simulink model "MyVhclOperator_RTW"  (Simulink 7.5)
settings: Solver=ode1  SolverMode=SingleTasking  StartTime=0.0  StopTime=inf  FixedStep=0.001  RelTol=1e-3
PreLoadFcn:
  | vehicle = 'Car'; if ~length(which('cmcmd')), cmenv; end
  | MyVhclOperator_RTW_bus
InitFcn:
  | vehicle = 'Car'; if ~length(which('cmcmd')), cmenv; end
  | MyVhclOperator_RTW_bus
undefined symbols (not defined in the file or in its folder): OperationFinished, Phase, SteerAng, VCBus
libraries: simulink x45
(part 2 of 3)

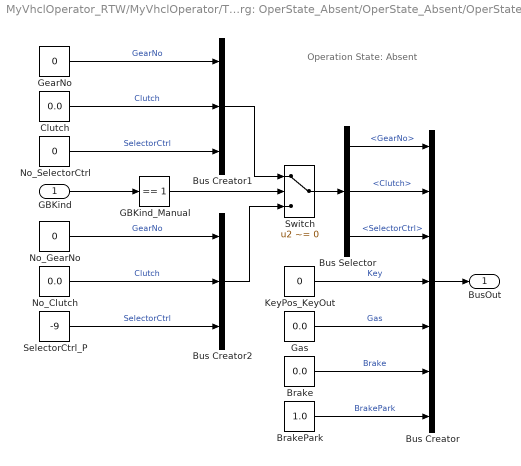
== system MyVhclOperator_RTW/MyVhclOperator/Trg: OperState_Absent/OperState_Absent/OperState: Absent ==
  note: Operation State:
      | Absent
  GBKind : Inport  OutDataType=fixdt(1, 16)  OutScaling=2^0
  Brake : Constant  Value=0.0  OutDataType=fixdt(1, 16)  OutScaling=2^0
  BrakePark : Constant  Value=1.0  OutDataType=fixdt(1, 16)  OutScaling=2^0
  Bus Creator : BusCreator  Inputs=7
  Bus Creator1 : BusCreator  Inputs=3
  Bus Creator2 : BusCreator  Inputs=3
  Bus Selector : BusSelector  OutputSignals=GearNo,Clutch,SelectorCtrl
  Clutch : Constant  Value=0.0  OutDataType=fixdt(1, 16)  OutScaling=2^0
  GBKind_Manual : simulink/Logic and Bit Operations/Compare To Constant  SystemSampleTime=-1  relop===  const=1  LogicOutDataTypeMode=uint8
  Gas : Constant  Value=0.0  OutDataType=fixdt(1, 16)  OutScaling=2^0
  GearNo : Constant  Value=0  OutDataType=fixdt(1, 16)  OutScaling=2^0
  KeyPos_KeyOut : Constant  Value=0  OutDataType=fixdt(1, 16)  OutScaling=2^0
  No_Clutch : Constant  Value=0.0  OutDataType=fixdt(1, 16)  OutScaling=2^0
  No_GearNo : Constant  Value=0  OutDataType=fixdt(1, 16)  OutScaling=2^0
  No_SelectorCtrl : Constant  Value=0  OutDataType=fixdt(1, 16)  OutScaling=2^0
  SelectorCtrl_P : Constant  Value=-9  OutDataType=fixdt(1, 16)  OutScaling=2^0
  Switch : Switch  Criteria=u2 ~= 0  OutDataType=fixdt(1, 16)  OutScaling=2^0
  BusOut : Outport  OutDataType=fixdt(1, 16)  OutScaling=2^0
  wires:
  GBKind_Manual/1 -> Switch/2
  GBKind/1 -> GBKind_Manual/1
  Bus Creator2/1 -> Switch/3
  SelectorCtrl_P/1 -> Bus Creator2/3  "SelectorCtrl"
  No_Clutch/1 -> Bus Creator2/2  "Clutch"
  No_GearNo/1 -> Bus Creator2/1  "GearNo"
  No_SelectorCtrl/1 -> Bus Creator1/3  "SelectorCtrl"
  Clutch/1 -> Bus Creator1/2  "Clutch"
  GearNo/1 -> Bus Creator1/1  "GearNo"
  Bus Creator1/1 -> Switch/1
  Switch/1 -> Bus Selector/1
  BrakePark/1 -> Bus Creator/7  "BrakePark"
  Brake/1 -> Bus Creator/6  "Brake"
  Gas/1 -> Bus Creator/5  "Gas"
  KeyPos_KeyOut/1 -> Bus Creator/4  "Key"
  Bus Selector/3 -> Bus Creator/3  "<SelectorCtrl>"
  Bus Selector/2 -> Bus Creator/2  "<Clutch>"
  Bus Selector/1 -> Bus Creator/1  "<GearNo>"
  Bus Creator/1 -> BusOut/1

== system MyVhclOperator_RTW/MyVhclOperator/Trg: OperState_Absent/OperState_Driving/Drive2Off ==
  note: Drive2Off
  BusIn : Inport  OutDataType=fixdt(1, 16)  OutScaling=2^0
  Active Brake : Subsystem  TreatAsAtomicUnit=on
  Brake to standstill? : Subsystem  TreatAsAtomicUnit=on
  Bus Selector : BusSelector  OutputSignals=Phase
  BusIn_Copy : InportShadow  Port=1  OutDataType=fixdt(1, 16)  OutScaling=2^0
  Key PowerOff : Subsystem  TreatAsAtomicUnit=on
  Merge : Merge  Inputs=5
  Switch Case : SwitchCase  CaseConditions={0,1,2,3,4}  ShowDefaultCase=off
  Wait for PowerOff : Subsystem  TreatAsAtomicUnit=on
  Wait until Standstill : Subsystem  TreatAsAtomicUnit=on
  BusOut : Outport  OutDataType=fixdt(1, 16)  OutScaling=2^0
  wires:
  Bus Selector/1 -> Switch Case/1  "<Phase>"
  Wait for PowerOff/1(BusOut) -> Merge/5
  Key PowerOff/1(BusOut) -> Merge/4
  Wait until Standstill/1(BusOut) -> Merge/3
  Active Brake/1(BusOut) -> Merge/2
  Brake to standstill?/1(BusOut) -> Merge/1
  BusIn_Copy/1 -> Brake to standstill?/1(BusIn), Active Brake/1(BusIn), Wait until Standstill/1(BusIn), Key PowerOff/1(BusIn), Wait for PowerOff/1(BusIn)
  Switch Case/5 -> Wait for PowerOff/Action
  Switch Case/4 -> Key PowerOff/Action
  Switch Case/3 -> Wait until Standstill/Action
  Merge/1 -> BusOut/1
  Switch Case/2 -> Active Brake/Action
  Switch Case/1 -> Brake to standstill?/Action
  BusIn/1 -> Bus Selector/1

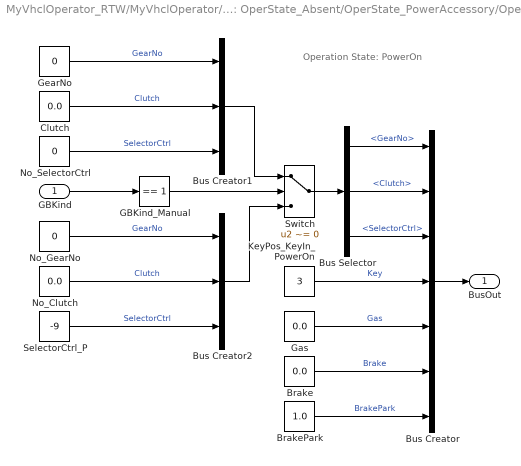
== system MyVhclOperator_RTW/MyVhclOperator/Trg: OperState_Absent/OperState_PowerAccessory/OperState: PowerOn ==
  note: Operation State:
      | PowerOn
  GBKind : Inport  OutDataType=fixdt(1, 16)  OutScaling=2^0
  Brake : Constant  Value=0.0  OutDataType=fixdt(1, 16)  OutScaling=2^0
  BrakePark : Constant  Value=1.0  OutDataType=fixdt(1, 16)  OutScaling=2^0
  Bus Creator : BusCreator  Inputs=7
  Bus Creator1 : BusCreator  Inputs=3
  Bus Creator2 : BusCreator  Inputs=3
  Bus Selector : BusSelector  OutputSignals=GearNo,Clutch,SelectorCtrl
  Clutch : Constant  Value=0.0  OutDataType=fixdt(1, 16)  OutScaling=2^0
  GBKind_Manual : simulink/Logic and Bit Operations/Compare To Constant  SystemSampleTime=-1  relop===  const=1  LogicOutDataTypeMode=uint8
  Gas : Constant  Value=0.0  OutDataType=fixdt(1, 16)  OutScaling=2^0
  GearNo : Constant  Value=0  OutDataType=fixdt(1, 16)  OutScaling=2^0
  KeyPos_KeyIn_PowerOn : Constant  Value=3  OutDataType=fixdt(1, 16)  OutScaling=2^0
  No_Clutch : Constant  Value=0.0  OutDataType=fixdt(1, 16)  OutScaling=2^0
  No_GearNo : Constant  Value=0  OutDataType=fixdt(1, 16)  OutScaling=2^0
  No_SelectorCtrl : Constant  Value=0  OutDataType=fixdt(1, 16)  OutScaling=2^0
  SelectorCtrl_P : Constant  Value=-9  OutDataType=fixdt(1, 16)  OutScaling=2^0
  Switch : Switch  Criteria=u2 ~= 0  OutDataType=fixdt(1, 16)  OutScaling=2^0
  BusOut : Outport  OutDataType=fixdt(1, 16)  OutScaling=2^0
  wires:
  GBKind_Manual/1 -> Switch/2
  GBKind/1 -> GBKind_Manual/1
  Bus Creator2/1 -> Switch/3
  SelectorCtrl_P/1 -> Bus Creator2/3  "SelectorCtrl"
  No_Clutch/1 -> Bus Creator2/2  "Clutch"
  No_GearNo/1 -> Bus Creator2/1  "GearNo"
  No_SelectorCtrl/1 -> Bus Creator1/3  "SelectorCtrl"
  Clutch/1 -> Bus Creator1/2  "Clutch"
  GearNo/1 -> Bus Creator1/1  "GearNo"
  Bus Creator1/1 -> Switch/1
  Switch/1 -> Bus Selector/1
  BrakePark/1 -> Bus Creator/7  "BrakePark"
  Brake/1 -> Bus Creator/6  "Brake"
  Gas/1 -> Bus Creator/5  "Gas"
  KeyPos_KeyIn_PowerOn/1 -> Bus Creator/4  "Key"
  Bus Selector/3 -> Bus Creator/3  "<SelectorCtrl>"
  Bus Selector/2 -> Bus Creator/2  "<Clutch>"
  Bus Selector/1 -> Bus Creator/1  "<GearNo>"
  Bus Creator/1 -> BusOut/1

== system MyVhclOperator_RTW/MyVhclOperator/Trg: OperState_Absent/OperState_PowerAccessory/SetOutputAndWait ==
  PhaseIn : Inport  OutDataType=fixdt(1, 16)  OutScaling=2^0
  Add : Sum  OutDataType=fixdt(1, 16)  OutScaling=2^-10
  Compare To Constant : simulink/Logic and Bit Operations/Compare To Constant  SystemSampleTime=-1  relop===  const=0  LogicOutDataTypeMode=uint8
  Constant : Constant  OutDataType=fixdt(1, 16)  OutScaling=2^0
  Switch : Switch  Criteria=u2 ~= 0  OutDataType=fixdt(1, 16)  OutScaling=2^0
  PhaseOut : Outport  OutDataType=fixdt(1, 16)  OutScaling=2^0
  wires:
  Constant/1 -> Add/1
  Add/1 -> Switch/1
  Compare To Constant/1 -> Switch/2
  PhaseIn/1 -> Add/2, Switch/3, Compare To Constant/1
  Switch/1 -> PhaseOut/1

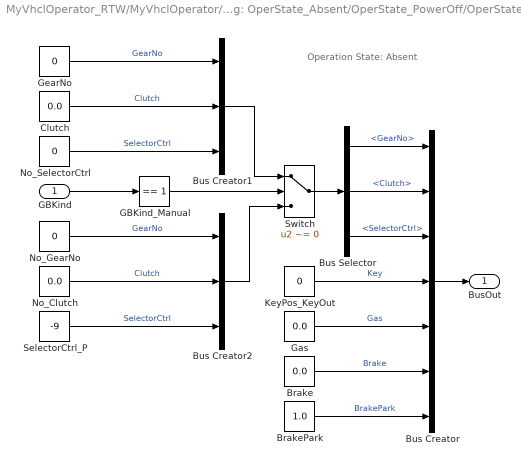
== system MyVhclOperator_RTW/MyVhclOperator/Trg: OperState_Absent/OperState_PowerOff/OperState: Absent ==
  note: Operation State:
      | Absent
  GBKind : Inport  OutDataType=fixdt(1, 16)  OutScaling=2^0
  Brake : Constant  Value=0.0  OutDataType=fixdt(1, 16)  OutScaling=2^0
  BrakePark : Constant  Value=1.0  OutDataType=fixdt(1, 16)  OutScaling=2^0
  Bus Creator : BusCreator  Inputs=7
  Bus Creator1 : BusCreator  Inputs=3
  Bus Creator2 : BusCreator  Inputs=3
  Bus Selector : BusSelector  OutputSignals=GearNo,Clutch,SelectorCtrl
  Clutch : Constant  Value=0.0  OutDataType=fixdt(1, 16)  OutScaling=2^0
  GBKind_Manual : simulink/Logic and Bit Operations/Compare To Constant  SystemSampleTime=-1  relop===  const=1  LogicOutDataTypeMode=uint8
  Gas : Constant  Value=0.0  OutDataType=fixdt(1, 16)  OutScaling=2^0
  GearNo : Constant  Value=0  OutDataType=fixdt(1, 16)  OutScaling=2^0
  KeyPos_KeyOut : Constant  Value=0  OutDataType=fixdt(1, 16)  OutScaling=2^0
  No_Clutch : Constant  Value=0.0  OutDataType=fixdt(1, 16)  OutScaling=2^0
  No_GearNo : Constant  Value=0  OutDataType=fixdt(1, 16)  OutScaling=2^0
  No_SelectorCtrl : Constant  Value=0  OutDataType=fixdt(1, 16)  OutScaling=2^0
  SelectorCtrl_P : Constant  Value=-9  OutDataType=fixdt(1, 16)  OutScaling=2^0
  Switch : Switch  Criteria=u2 ~= 0  OutDataType=fixdt(1, 16)  OutScaling=2^0
  BusOut : Outport  OutDataType=fixdt(1, 16)  OutScaling=2^0
  wires:
  GBKind_Manual/1 -> Switch/2
  GBKind/1 -> GBKind_Manual/1
  Bus Creator2/1 -> Switch/3
  SelectorCtrl_P/1 -> Bus Creator2/3  "SelectorCtrl"
  No_Clutch/1 -> Bus Creator2/2  "Clutch"
  No_GearNo/1 -> Bus Creator2/1  "GearNo"
  No_SelectorCtrl/1 -> Bus Creator1/3  "SelectorCtrl"
  Clutch/1 -> Bus Creator1/2  "Clutch"
  GearNo/1 -> Bus Creator1/1  "GearNo"
  Bus Creator1/1 -> Switch/1
  Switch/1 -> Bus Selector/1
  BrakePark/1 -> Bus Creator/7  "BrakePark"
  Brake/1 -> Bus Creator/6  "Brake"
  Gas/1 -> Bus Creator/5  "Gas"
  KeyPos_KeyOut/1 -> Bus Creator/4  "Key"
  Bus Selector/3 -> Bus Creator/3  "<SelectorCtrl>"
  Bus Selector/2 -> Bus Creator/2  "<Clutch>"
  Bus Selector/1 -> Bus Creator/1  "<GearNo>"
  Bus Creator/1 -> BusOut/1

== system MyVhclOperator_RTW/MyVhclOperator/Trg: OperState_Absent/OperState_PowerOff/SetOutputAndWait ==
  PhaseIn : Inport  OutDataType=fixdt(1, 16)  OutScaling=2^0
  Add : Sum  OutDataType=fixdt(1, 16)  OutScaling=2^-10
  Compare To Constant : simulink/Logic and Bit Operations/Compare To Constant  SystemSampleTime=-1  relop===  const=0  LogicOutDataTypeMode=uint8
  Constant : Constant  OutDataType=fixdt(1, 16)  OutScaling=2^0
  Switch : Switch  Criteria=u2 ~= 0  OutDataType=fixdt(1, 16)  OutScaling=2^0
  PhaseOut : Outport  OutDataType=fixdt(1, 16)  OutScaling=2^0
  wires:
  Constant/1 -> Add/1
  Add/1 -> Switch/1
  Compare To Constant/1 -> Switch/2
  PhaseIn/1 -> Add/2, Switch/3, Compare To Constant/1
  Switch/1 -> PhaseOut/1

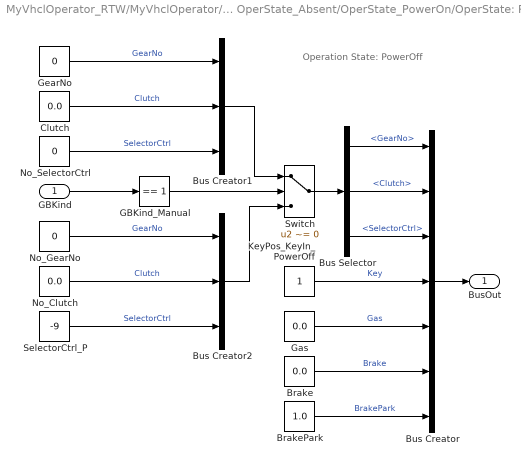
== system MyVhclOperator_RTW/MyVhclOperator/Trg: OperState_Absent/OperState_PowerOn/OperState: PowerOff ==
  note: Operation State:
      | PowerOff
  GBKind : Inport  OutDataType=fixdt(1, 16)  OutScaling=2^0
  Brake : Constant  Value=0.0  OutDataType=fixdt(1, 16)  OutScaling=2^0
  BrakePark : Constant  Value=1.0  OutDataType=fixdt(1, 16)  OutScaling=2^0
  Bus Creator : BusCreator  Inputs=7
  Bus Creator1 : BusCreator  Inputs=3
  Bus Creator2 : BusCreator  Inputs=3
  Bus Selector : BusSelector  OutputSignals=GearNo,Clutch,SelectorCtrl
  Clutch : Constant  Value=0.0  OutDataType=fixdt(1, 16)  OutScaling=2^0
  GBKind_Manual : simulink/Logic and Bit Operations/Compare To Constant  SystemSampleTime=-1  relop===  const=1  LogicOutDataTypeMode=uint8
  Gas : Constant  Value=0.0  OutDataType=fixdt(1, 16)  OutScaling=2^0
  GearNo : Constant  Value=0  OutDataType=fixdt(1, 16)  OutScaling=2^0
  KeyPos_KeyIn_PowerOff : Constant  OutDataType=fixdt(1, 16)  OutScaling=2^0
  No_Clutch : Constant  Value=0.0  OutDataType=fixdt(1, 16)  OutScaling=2^0
  No_GearNo : Constant  Value=0  OutDataType=fixdt(1, 16)  OutScaling=2^0
  No_SelectorCtrl : Constant  Value=0  OutDataType=fixdt(1, 16)  OutScaling=2^0
  SelectorCtrl_P : Constant  Value=-9  OutDataType=fixdt(1, 16)  OutScaling=2^0
  Switch : Switch  Criteria=u2 ~= 0  OutDataType=fixdt(1, 16)  OutScaling=2^0
  BusOut : Outport  OutDataType=fixdt(1, 16)  OutScaling=2^0
  wires:
  GBKind_Manual/1 -> Switch/2
  GBKind/1 -> GBKind_Manual/1
  Bus Creator2/1 -> Switch/3
  SelectorCtrl_P/1 -> Bus Creator2/3  "SelectorCtrl"
  No_Clutch/1 -> Bus Creator2/2  "Clutch"
  No_GearNo/1 -> Bus Creator2/1  "GearNo"
  No_SelectorCtrl/1 -> Bus Creator1/3  "SelectorCtrl"
  Clutch/1 -> Bus Creator1/2  "Clutch"
  GearNo/1 -> Bus Creator1/1  "GearNo"
  Bus Creator1/1 -> Switch/1
  Switch/1 -> Bus Selector/1
  BrakePark/1 -> Bus Creator/7  "BrakePark"
  Brake/1 -> Bus Creator/6  "Brake"
  Gas/1 -> Bus Creator/5  "Gas"
  KeyPos_KeyIn_PowerOff/1 -> Bus Creator/4  "Key"
  Bus Selector/3 -> Bus Creator/3  "<SelectorCtrl>"
  Bus Selector/2 -> Bus Creator/2  "<Clutch>"
  Bus Selector/1 -> Bus Creator/1  "<GearNo>"
  Bus Creator/1 -> BusOut/1

== system MyVhclOperator_RTW/MyVhclOperator/Trg: OperState_Absent/OperState_PowerOn/SetOutputAndWait ==
  PhaseIn : Inport  OutDataType=fixdt(1, 16)  OutScaling=2^0
  Add : Sum  OutDataType=fixdt(1, 16)  OutScaling=2^-10
  Compare To Constant : simulink/Logic and Bit Operations/Compare To Constant  SystemSampleTime=-1  relop===  const=0  LogicOutDataTypeMode=uint8
  Constant : Constant  OutDataType=fixdt(1, 16)  OutScaling=2^0
  Switch : Switch  Criteria=u2 ~= 0  OutDataType=fixdt(1, 16)  OutScaling=2^0
  PhaseOut : Outport  OutDataType=fixdt(1, 16)  OutScaling=2^0
  wires:
  Switch/1 -> PhaseOut/1
  PhaseIn/1 -> Compare To Constant/1, Switch/3, Add/2
  Compare To Constant/1 -> Switch/2
  Add/1 -> Switch/1
  Constant/1 -> Add/1

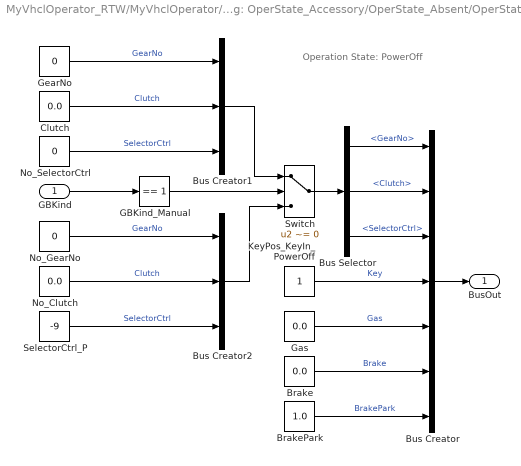
== system MyVhclOperator_RTW/MyVhclOperator/Trg: OperState_Accessory/OperState_Absent/OperState: PowerOff ==
  note: Operation State:
      | PowerOff
  GBKind : Inport  OutDataType=fixdt(1, 16)  OutScaling=2^0
  Brake : Constant  Value=0.0  OutDataType=fixdt(1, 16)  OutScaling=2^0
  BrakePark : Constant  Value=1.0  OutDataType=fixdt(1, 16)  OutScaling=2^0
  Bus Creator : BusCreator  Inputs=7
  Bus Creator1 : BusCreator  Inputs=3
  Bus Creator2 : BusCreator  Inputs=3
  Bus Selector : BusSelector  OutputSignals=GearNo,Clutch,SelectorCtrl
  Clutch : Constant  Value=0.0  OutDataType=fixdt(1, 16)  OutScaling=2^0
  GBKind_Manual : simulink/Logic and Bit Operations/Compare To Constant  SystemSampleTime=-1  relop===  const=1  LogicOutDataTypeMode=uint8
  Gas : Constant  Value=0.0  OutDataType=fixdt(1, 16)  OutScaling=2^0
  GearNo : Constant  Value=0  OutDataType=fixdt(1, 16)  OutScaling=2^0
  KeyPos_KeyIn_PowerOff : Constant  OutDataType=fixdt(1, 16)  OutScaling=2^0
  No_Clutch : Constant  Value=0.0  OutDataType=fixdt(1, 16)  OutScaling=2^0
  No_GearNo : Constant  Value=0  OutDataType=fixdt(1, 16)  OutScaling=2^0
  No_SelectorCtrl : Constant  Value=0  OutDataType=fixdt(1, 16)  OutScaling=2^0
  SelectorCtrl_P : Constant  Value=-9  OutDataType=fixdt(1, 16)  OutScaling=2^0
  Switch : Switch  Criteria=u2 ~= 0  OutDataType=fixdt(1, 16)  OutScaling=2^0
  BusOut : Outport  OutDataType=fixdt(1, 16)  OutScaling=2^0
  wires:
  Bus Creator/1 -> BusOut/1
  Bus Selector/1 -> Bus Creator/1  "<GearNo>"
  Bus Selector/2 -> Bus Creator/2  "<Clutch>"
  Bus Selector/3 -> Bus Creator/3  "<SelectorCtrl>"
  KeyPos_KeyIn_PowerOff/1 -> Bus Creator/4  "Key"
  Gas/1 -> Bus Creator/5  "Gas"
  Brake/1 -> Bus Creator/6  "Brake"
  BrakePark/1 -> Bus Creator/7  "BrakePark"
  Switch/1 -> Bus Selector/1
  Bus Creator1/1 -> Switch/1
  GearNo/1 -> Bus Creator1/1  "GearNo"
  Clutch/1 -> Bus Creator1/2  "Clutch"
  No_SelectorCtrl/1 -> Bus Creator1/3  "SelectorCtrl"
  No_GearNo/1 -> Bus Creator2/1  "GearNo"
  No_Clutch/1 -> Bus Creator2/2  "Clutch"
  SelectorCtrl_P/1 -> Bus Creator2/3  "SelectorCtrl"
  Bus Creator2/1 -> Switch/3
  GBKind/1 -> GBKind_Manual/1
  GBKind_Manual/1 -> Switch/2

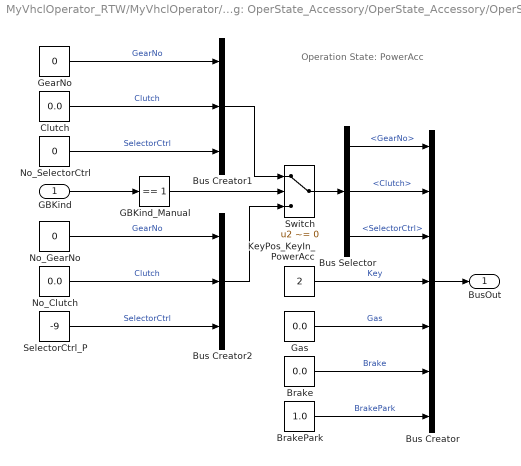
== system MyVhclOperator_RTW/MyVhclOperator/Trg: OperState_Accessory/OperState_Accessory/OperState: PowerAcc ==
  note: Operation State:
      | PowerAcc
  GBKind : Inport  OutDataType=fixdt(1, 16)  OutScaling=2^0
  Brake : Constant  Value=0.0  OutDataType=fixdt(1, 16)  OutScaling=2^0
  BrakePark : Constant  Value=1.0  OutDataType=fixdt(1, 16)  OutScaling=2^0
  Bus Creator : BusCreator  Inputs=7
  Bus Creator1 : BusCreator  Inputs=3
  Bus Creator2 : BusCreator  Inputs=3
  Bus Selector : BusSelector  OutputSignals=GearNo,Clutch,SelectorCtrl
  Clutch : Constant  Value=0.0  OutDataType=fixdt(1, 16)  OutScaling=2^0
  GBKind_Manual : simulink/Logic and Bit Operations/Compare To Constant  SystemSampleTime=-1  relop===  const=1  LogicOutDataTypeMode=uint8
  Gas : Constant  Value=0.0  OutDataType=fixdt(1, 16)  OutScaling=2^0
  GearNo : Constant  Value=0  OutDataType=fixdt(1, 16)  OutScaling=2^0
  KeyPos_KeyIn_PowerAcc : Constant  Value=2  OutDataType=fixdt(1, 16)  OutScaling=2^0
  No_Clutch : Constant  Value=0.0  OutDataType=fixdt(1, 16)  OutScaling=2^0
  No_GearNo : Constant  Value=0  OutDataType=fixdt(1, 16)  OutScaling=2^0
  No_SelectorCtrl : Constant  Value=0  OutDataType=fixdt(1, 16)  OutScaling=2^0
  SelectorCtrl_P : Constant  Value=-9  OutDataType=fixdt(1, 16)  OutScaling=2^0
  Switch : Switch  Criteria=u2 ~= 0  OutDataType=fixdt(1, 16)  OutScaling=2^0
  BusOut : Outport  OutDataType=fixdt(1, 16)  OutScaling=2^0
  wires:
  GBKind_Manual/1 -> Switch/2
  GBKind/1 -> GBKind_Manual/1
  Bus Creator2/1 -> Switch/3
  SelectorCtrl_P/1 -> Bus Creator2/3  "SelectorCtrl"
  No_Clutch/1 -> Bus Creator2/2  "Clutch"
  No_GearNo/1 -> Bus Creator2/1  "GearNo"
  No_SelectorCtrl/1 -> Bus Creator1/3  "SelectorCtrl"
  Clutch/1 -> Bus Creator1/2  "Clutch"
  GearNo/1 -> Bus Creator1/1  "GearNo"
  Bus Creator1/1 -> Switch/1
  Switch/1 -> Bus Selector/1
  BrakePark/1 -> Bus Creator/7  "BrakePark"
  Brake/1 -> Bus Creator/6  "Brake"
  Gas/1 -> Bus Creator/5  "Gas"
  KeyPos_KeyIn_PowerAcc/1 -> Bus Creator/4  "Key"
  Bus Selector/3 -> Bus Creator/3  "<SelectorCtrl>"
  Bus Selector/2 -> Bus Creator/2  "<Clutch>"
  Bus Selector/1 -> Bus Creator/1  "<GearNo>"
  Bus Creator/1 -> BusOut/1

== system MyVhclOperator_RTW/MyVhclOperator/Trg: OperState_Accessory/OperState_Driving/Drive2Off ==
  note: Drive2Off
  BusIn : Inport  OutDataType=fixdt(1, 16)  OutScaling=2^0
  Active Brake : Subsystem  TreatAsAtomicUnit=on
  Brake to standstill? : Subsystem  TreatAsAtomicUnit=on
  Bus Selector : BusSelector  OutputSignals=Phase
  BusIn_Copy : InportShadow  Port=1  OutDataType=fixdt(1, 16)  OutScaling=2^0
  Key PowerOff : Subsystem  TreatAsAtomicUnit=on
  Merge : Merge  Inputs=5
  Switch Case : SwitchCase  CaseConditions={0,1,2,3,4}  ShowDefaultCase=off
  Wait for PowerOff : Subsystem  TreatAsAtomicUnit=on
  Wait until Standstill : Subsystem  TreatAsAtomicUnit=on
  BusOut : Outport  OutDataType=fixdt(1, 16)  OutScaling=2^0
  wires:
  Bus Selector/1 -> Switch Case/1  "<Phase>"
  Wait for PowerOff/1(BusOut) -> Merge/5
  Key PowerOff/1(BusOut) -> Merge/4
  Wait until Standstill/1(BusOut) -> Merge/3
  Active Brake/1(BusOut) -> Merge/2
  Brake to standstill?/1(BusOut) -> Merge/1
  BusIn_Copy/1 -> Brake to standstill?/1(BusIn), Active Brake/1(BusIn), Wait until Standstill/1(BusIn), Key PowerOff/1(BusIn), Wait for PowerOff/1(BusIn)
  Switch Case/5 -> Wait for PowerOff/Action
  Switch Case/4 -> Key PowerOff/Action
  Switch Case/3 -> Wait until Standstill/Action
  Merge/1 -> BusOut/1
  Switch Case/2 -> Active Brake/Action
  Switch Case/1 -> Brake to standstill?/Action
  BusIn/1 -> Bus Selector/1

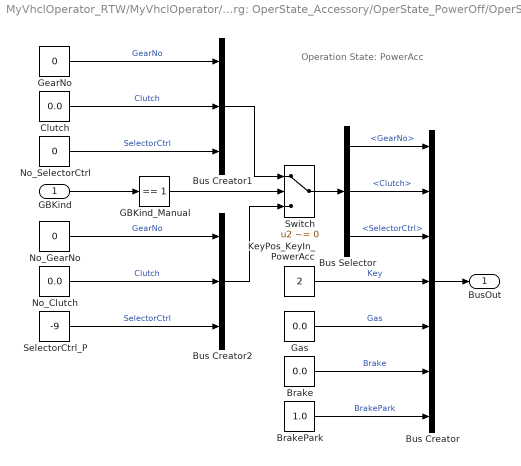
== system MyVhclOperator_RTW/MyVhclOperator/Trg: OperState_Accessory/OperState_PowerOff/OperState: PowerAcc ==
  note: Operation State:
      | PowerAcc
  GBKind : Inport  OutDataType=fixdt(1, 16)  OutScaling=2^0
  Brake : Constant  Value=0.0  OutDataType=fixdt(1, 16)  OutScaling=2^0
  BrakePark : Constant  Value=1.0  OutDataType=fixdt(1, 16)  OutScaling=2^0
  Bus Creator : BusCreator  Inputs=7
  Bus Creator1 : BusCreator  Inputs=3
  Bus Creator2 : BusCreator  Inputs=3
  Bus Selector : BusSelector  OutputSignals=GearNo,Clutch,SelectorCtrl
  Clutch : Constant  Value=0.0  OutDataType=fixdt(1, 16)  OutScaling=2^0
  GBKind_Manual : simulink/Logic and Bit Operations/Compare To Constant  SystemSampleTime=-1  relop===  const=1  LogicOutDataTypeMode=uint8
  Gas : Constant  Value=0.0  OutDataType=fixdt(1, 16)  OutScaling=2^0
  GearNo : Constant  Value=0  OutDataType=fixdt(1, 16)  OutScaling=2^0
  KeyPos_KeyIn_PowerAcc : Constant  Value=2  OutDataType=fixdt(1, 16)  OutScaling=2^0
  No_Clutch : Constant  Value=0.0  OutDataType=fixdt(1, 16)  OutScaling=2^0
  No_GearNo : Constant  Value=0  OutDataType=fixdt(1, 16)  OutScaling=2^0
  No_SelectorCtrl : Constant  Value=0  OutDataType=fixdt(1, 16)  OutScaling=2^0
  SelectorCtrl_P : Constant  Value=-9  OutDataType=fixdt(1, 16)  OutScaling=2^0
  Switch : Switch  Criteria=u2 ~= 0  OutDataType=fixdt(1, 16)  OutScaling=2^0
  BusOut : Outport  OutDataType=fixdt(1, 16)  OutScaling=2^0
  wires:
  GBKind_Manual/1 -> Switch/2
  GBKind/1 -> GBKind_Manual/1
  Bus Creator2/1 -> Switch/3
  SelectorCtrl_P/1 -> Bus Creator2/3  "SelectorCtrl"
  No_Clutch/1 -> Bus Creator2/2  "Clutch"
  No_GearNo/1 -> Bus Creator2/1  "GearNo"
  No_SelectorCtrl/1 -> Bus Creator1/3  "SelectorCtrl"
  Clutch/1 -> Bus Creator1/2  "Clutch"
  GearNo/1 -> Bus Creator1/1  "GearNo"
  Bus Creator1/1 -> Switch/1
  Switch/1 -> Bus Selector/1
  BrakePark/1 -> Bus Creator/7  "BrakePark"
  Brake/1 -> Bus Creator/6  "Brake"
  Gas/1 -> Bus Creator/5  "Gas"
  KeyPos_KeyIn_PowerAcc/1 -> Bus Creator/4  "Key"
  Bus Selector/3 -> Bus Creator/3  "<SelectorCtrl>"
  Bus Selector/2 -> Bus Creator/2  "<Clutch>"
  Bus Selector/1 -> Bus Creator/1  "<GearNo>"
  Bus Creator/1 -> BusOut/1

== system MyVhclOperator_RTW/MyVhclOperator/Trg: OperState_Accessory/OperState_PowerOff/SetOutputAndWait ==
  PhaseIn : Inport  OutDataType=fixdt(1, 16)  OutScaling=2^0
  Add : Sum  OutDataType=fixdt(1, 16)  OutScaling=2^-10
  Compare To Constant : simulink/Logic and Bit Operations/Compare To Constant  SystemSampleTime=-1  relop===  const=0  LogicOutDataTypeMode=uint8
  Constant : Constant  OutDataType=fixdt(1, 16)  OutScaling=2^0
  Switch : Switch  Criteria=u2 ~= 0  OutDataType=fixdt(1, 16)  OutScaling=2^0
  PhaseOut : Outport  OutDataType=fixdt(1, 16)  OutScaling=2^0
  wires:
  Switch/1 -> PhaseOut/1
  PhaseIn/1 -> Compare To Constant/1, Switch/3, Add/2
  Compare To Constant/1 -> Switch/2
  Add/1 -> Switch/1
  Constant/1 -> Add/1

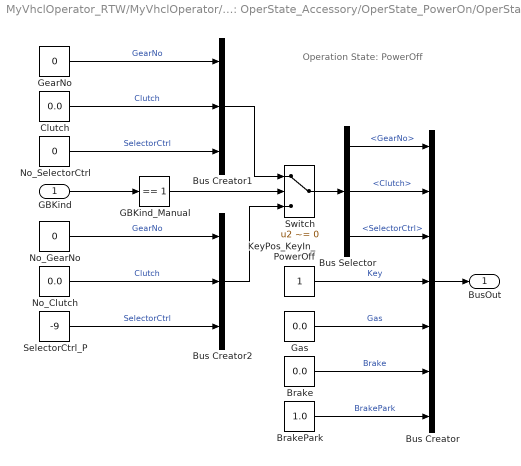
== system MyVhclOperator_RTW/MyVhclOperator/Trg: OperState_Accessory/OperState_PowerOn/OperState: PowerOff ==
  note: Operation State:
      | PowerOff
  GBKind : Inport  OutDataType=fixdt(1, 16)  OutScaling=2^0
  Brake : Constant  Value=0.0  OutDataType=fixdt(1, 16)  OutScaling=2^0
  BrakePark : Constant  Value=1.0  OutDataType=fixdt(1, 16)  OutScaling=2^0
  Bus Creator : BusCreator  Inputs=7
  Bus Creator1 : BusCreator  Inputs=3
  Bus Creator2 : BusCreator  Inputs=3
  Bus Selector : BusSelector  OutputSignals=GearNo,Clutch,SelectorCtrl
  Clutch : Constant  Value=0.0  OutDataType=fixdt(1, 16)  OutScaling=2^0
  GBKind_Manual : simulink/Logic and Bit Operations/Compare To Constant  SystemSampleTime=-1  relop===  const=1  LogicOutDataTypeMode=uint8
  Gas : Constant  Value=0.0  OutDataType=fixdt(1, 16)  OutScaling=2^0
  GearNo : Constant  Value=0  OutDataType=fixdt(1, 16)  OutScaling=2^0
  KeyPos_KeyIn_PowerOff : Constant  OutDataType=fixdt(1, 16)  OutScaling=2^0
  No_Clutch : Constant  Value=0.0  OutDataType=fixdt(1, 16)  OutScaling=2^0
  No_GearNo : Constant  Value=0  OutDataType=fixdt(1, 16)  OutScaling=2^0
  No_SelectorCtrl : Constant  Value=0  OutDataType=fixdt(1, 16)  OutScaling=2^0
  SelectorCtrl_P : Constant  Value=-9  OutDataType=fixdt(1, 16)  OutScaling=2^0
  Switch : Switch  Criteria=u2 ~= 0  OutDataType=fixdt(1, 16)  OutScaling=2^0
  BusOut : Outport  OutDataType=fixdt(1, 16)  OutScaling=2^0
  wires:
  GBKind_Manual/1 -> Switch/2
  GBKind/1 -> GBKind_Manual/1
  Bus Creator2/1 -> Switch/3
  SelectorCtrl_P/1 -> Bus Creator2/3  "SelectorCtrl"
  No_Clutch/1 -> Bus Creator2/2  "Clutch"
  No_GearNo/1 -> Bus Creator2/1  "GearNo"
  No_SelectorCtrl/1 -> Bus Creator1/3  "SelectorCtrl"
  Clutch/1 -> Bus Creator1/2  "Clutch"
  GearNo/1 -> Bus Creator1/1  "GearNo"
  Bus Creator1/1 -> Switch/1
  Switch/1 -> Bus Selector/1
  BrakePark/1 -> Bus Creator/7  "BrakePark"
  Brake/1 -> Bus Creator/6  "Brake"
  Gas/1 -> Bus Creator/5  "Gas"
  KeyPos_KeyIn_PowerOff/1 -> Bus Creator/4  "Key"
  Bus Selector/3 -> Bus Creator/3  "<SelectorCtrl>"
  Bus Selector/2 -> Bus Creator/2  "<Clutch>"
  Bus Selector/1 -> Bus Creator/1  "<GearNo>"
  Bus Creator/1 -> BusOut/1

== system MyVhclOperator_RTW/MyVhclOperator/Trg: OperState_Accessory/OperState_PowerOn/SetOutputAndWait ==
  PhaseIn : Inport  OutDataType=fixdt(1, 16)  OutScaling=2^0
  Add : Sum  OutDataType=fixdt(1, 16)  OutScaling=2^-10
  Compare To Constant : simulink/Logic and Bit Operations/Compare To Constant  SystemSampleTime=-1  relop===  const=0  LogicOutDataTypeMode=uint8
  Constant : Constant  OutDataType=fixdt(1, 16)  OutScaling=2^0
  Switch : Switch  Criteria=u2 ~= 0  OutDataType=fixdt(1, 16)  OutScaling=2^0
  PhaseOut : Outport  OutDataType=fixdt(1, 16)  OutScaling=2^0
  wires:
  Switch/1 -> PhaseOut/1
  PhaseIn/1 -> Compare To Constant/1, Switch/3, Add/2
  Compare To Constant/1 -> Switch/2
  Add/1 -> Switch/1
  Constant/1 -> Add/1

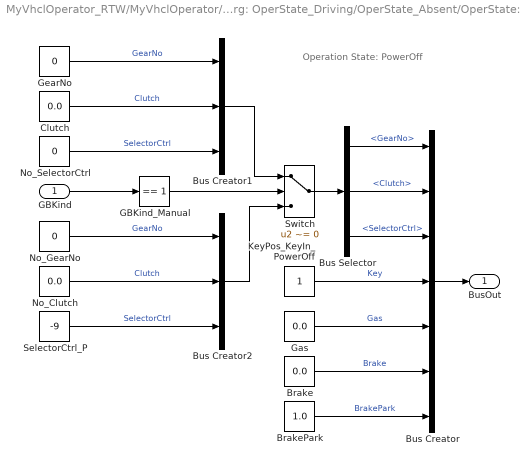
== system MyVhclOperator_RTW/MyVhclOperator/Trg: OperState_Driving/OperState_Absent/OperState: PowerOff ==
  note: Operation State:
      | PowerOff
  GBKind : Inport  OutDataType=fixdt(1, 16)  OutScaling=2^0
  Brake : Constant  Value=0.0  OutDataType=fixdt(1, 16)  OutScaling=2^0
  BrakePark : Constant  Value=1.0  OutDataType=fixdt(1, 16)  OutScaling=2^0
  Bus Creator : BusCreator  Inputs=7
  Bus Creator1 : BusCreator  Inputs=3
  Bus Creator2 : BusCreator  Inputs=3
  Bus Selector : BusSelector  OutputSignals=GearNo,Clutch,SelectorCtrl
  Clutch : Constant  Value=0.0  OutDataType=fixdt(1, 16)  OutScaling=2^0
  GBKind_Manual : simulink/Logic and Bit Operations/Compare To Constant  SystemSampleTime=-1  relop===  const=1  LogicOutDataTypeMode=uint8
  Gas : Constant  Value=0.0  OutDataType=fixdt(1, 16)  OutScaling=2^0
  GearNo : Constant  Value=0  OutDataType=fixdt(1, 16)  OutScaling=2^0
  KeyPos_KeyIn_PowerOff : Constant  OutDataType=fixdt(1, 16)  OutScaling=2^0
  No_Clutch : Constant  Value=0.0  OutDataType=fixdt(1, 16)  OutScaling=2^0
  No_GearNo : Constant  Value=0  OutDataType=fixdt(1, 16)  OutScaling=2^0
  No_SelectorCtrl : Constant  Value=0  OutDataType=fixdt(1, 16)  OutScaling=2^0
  SelectorCtrl_P : Constant  Value=-9  OutDataType=fixdt(1, 16)  OutScaling=2^0
  Switch : Switch  Criteria=u2 ~= 0  OutDataType=fixdt(1, 16)  OutScaling=2^0
  BusOut : Outport  OutDataType=fixdt(1, 16)  OutScaling=2^0
  wires:
  GBKind_Manual/1 -> Switch/2
  GBKind/1 -> GBKind_Manual/1
  Bus Creator2/1 -> Switch/3
  SelectorCtrl_P/1 -> Bus Creator2/3  "SelectorCtrl"
  No_Clutch/1 -> Bus Creator2/2  "Clutch"
  No_GearNo/1 -> Bus Creator2/1  "GearNo"
  No_SelectorCtrl/1 -> Bus Creator1/3  "SelectorCtrl"
  Clutch/1 -> Bus Creator1/2  "Clutch"
  GearNo/1 -> Bus Creator1/1  "GearNo"
  Bus Creator1/1 -> Switch/1
  Switch/1 -> Bus Selector/1
  BrakePark/1 -> Bus Creator/7  "BrakePark"
  Brake/1 -> Bus Creator/6  "Brake"
  Gas/1 -> Bus Creator/5  "Gas"
  KeyPos_KeyIn_PowerOff/1 -> Bus Creator/4  "Key"
  Bus Selector/3 -> Bus Creator/3  "<SelectorCtrl>"
  Bus Selector/2 -> Bus Creator/2  "<Clutch>"
  Bus Selector/1 -> Bus Creator/1  "<GearNo>"
  Bus Creator/1 -> BusOut/1

== system MyVhclOperator_RTW/MyVhclOperator/Trg: OperState_Driving/OperState_Driving/OperState: Driving ==
  note: Operation State:
      | Driving
  GBKind : Inport  OutDataType=fixdt(1, 16)  OutScaling=2^0
  Brake : Constant  Value=0.0  OutDataType=fixdt(1, 16)  OutScaling=2^0
  BrakePark : Constant  Value=0.0  OutDataType=fixdt(1, 16)  OutScaling=2^0
  Bus Creator : BusCreator  Inputs=7
  Bus Creator1 : BusCreator  Inputs=3
  Bus Creator2 : BusCreator  Inputs=3
  Bus Selector : BusSelector  OutputSignals=GearNo,Clutch,SelectorCtrl
  Clutch : Constant  Value=1.0  OutDataType=fixdt(1, 16)  OutScaling=2^0
  GBKind_Manual : simulink/Logic and Bit Operations/Compare To Constant  SystemSampleTime=-1  relop===  const=1  LogicOutDataTypeMode=uint8
  Gas : Constant  Value=0.0  OutDataType=fixdt(1, 16)  OutScaling=2^0
  GearNo : Constant  OutDataType=fixdt(1, 16)  OutScaling=2^0
  KeyPos_KeyIn_PowerOn : Constant  Value=3  OutDataType=fixdt(1, 16)  OutScaling=2^0
  No_Clutch : Constant  Value=0.0  OutDataType=fixdt(1, 16)  OutScaling=2^0
  No_GearNo : Constant  Value=0  OutDataType=fixdt(1, 16)  OutScaling=2^0
  No_SelectorCtrl : Constant  Value=0  OutDataType=fixdt(1, 16)  OutScaling=2^0
  SelectorCtrl_D : Constant  OutDataType=fixdt(1, 16)  OutScaling=2^0
  Switch : Switch  Criteria=u2 ~= 0  OutDataType=fixdt(1, 16)  OutScaling=2^0
  BusOut : Outport  OutDataType=fixdt(1, 16)  OutScaling=2^0
  wires:
  GBKind_Manual/1 -> Switch/2
  GBKind/1 -> GBKind_Manual/1
  Bus Creator2/1 -> Switch/3
  SelectorCtrl_D/1 -> Bus Creator2/3  "SelectorCtrl"
  No_Clutch/1 -> Bus Creator2/2  "Clutch"
  No_GearNo/1 -> Bus Creator2/1  "GearNo"
  No_SelectorCtrl/1 -> Bus Creator1/3  "SelectorCtrl"
  Clutch/1 -> Bus Creator1/2  "Clutch"
  GearNo/1 -> Bus Creator1/1  "GearNo"
  Bus Creator1/1 -> Switch/1
  Switch/1 -> Bus Selector/1
  BrakePark/1 -> Bus Creator/7  "BrakePark"
  Brake/1 -> Bus Creator/6  "Brake"
  Gas/1 -> Bus Creator/5  "Gas"
  KeyPos_KeyIn_PowerOn/1 -> Bus Creator/4  "Key"
  Bus Selector/3 -> Bus Creator/3  "<SelectorCtrl>"
  Bus Selector/2 -> Bus Creator/2  "<Clutch>"
  Bus Selector/1 -> Bus Creator/1  "<GearNo>"
  Bus Creator/1 -> BusOut/1

== system MyVhclOperator_RTW/MyVhclOperator/Trg: OperState_Driving/OperState_PowerAccessory/OperState: PowerOn ==
  note: Operation State:
      | PowerOn
  GBKind : Inport  OutDataType=fixdt(1, 16)  OutScaling=2^0
  Brake : Constant  Value=0.0  OutDataType=fixdt(1, 16)  OutScaling=2^0
  BrakePark : Constant  Value=1.0  OutDataType=fixdt(1, 16)  OutScaling=2^0
  Bus Creator : BusCreator  Inputs=7
  Bus Creator1 : BusCreator  Inputs=3
  Bus Creator2 : BusCreator  Inputs=3
  Bus Selector : BusSelector  OutputSignals=GearNo,Clutch,SelectorCtrl
  Clutch : Constant  Value=0.0  OutDataType=fixdt(1, 16)  OutScaling=2^0
  GBKind_Manual : simulink/Logic and Bit Operations/Compare To Constant  SystemSampleTime=-1  relop===  const=1  LogicOutDataTypeMode=uint8
  Gas : Constant  Value=0.0  OutDataType=fixdt(1, 16)  OutScaling=2^0
  GearNo : Constant  Value=0  OutDataType=fixdt(1, 16)  OutScaling=2^0
  KeyPos_KeyIn_PowerOn : Constant  Value=3  OutDataType=fixdt(1, 16)  OutScaling=2^0
  No_Clutch : Constant  Value=0.0  OutDataType=fixdt(1, 16)  OutScaling=2^0
  No_GearNo : Constant  Value=0  OutDataType=fixdt(1, 16)  OutScaling=2^0
  No_SelectorCtrl : Constant  Value=0  OutDataType=fixdt(1, 16)  OutScaling=2^0
  SelectorCtrl_P : Constant  Value=-9  OutDataType=fixdt(1, 16)  OutScaling=2^0
  Switch : Switch  Criteria=u2 ~= 0  OutDataType=fixdt(1, 16)  OutScaling=2^0
  BusOut : Outport  OutDataType=fixdt(1, 16)  OutScaling=2^0
  wires:
  Bus Creator/1 -> BusOut/1
  Bus Selector/1 -> Bus Creator/1  "<GearNo>"
  Bus Selector/2 -> Bus Creator/2  "<Clutch>"
  Bus Selector/3 -> Bus Creator/3  "<SelectorCtrl>"
  KeyPos_KeyIn_PowerOn/1 -> Bus Creator/4  "Key"
  Gas/1 -> Bus Creator/5  "Gas"
  Brake/1 -> Bus Creator/6  "Brake"
  BrakePark/1 -> Bus Creator/7  "BrakePark"
  Switch/1 -> Bus Selector/1
  Bus Creator1/1 -> Switch/1
  GearNo/1 -> Bus Creator1/1  "GearNo"
  Clutch/1 -> Bus Creator1/2  "Clutch"
  No_SelectorCtrl/1 -> Bus Creator1/3  "SelectorCtrl"
  No_GearNo/1 -> Bus Creator2/1  "GearNo"
  No_Clutch/1 -> Bus Creator2/2  "Clutch"
  SelectorCtrl_P/1 -> Bus Creator2/3  "SelectorCtrl"
  Bus Creator2/1 -> Switch/3
  GBKind/1 -> GBKind_Manual/1
  GBKind_Manual/1 -> Switch/2

== system MyVhclOperator_RTW/MyVhclOperator/Trg: OperState_Driving/OperState_PowerAccessory/SetOutputAndWait ==
  PhaseIn : Inport  OutDataType=fixdt(1, 16)  OutScaling=2^0
  Add : Sum  OutDataType=fixdt(1, 16)  OutScaling=2^-10
  Compare To Constant : simulink/Logic and Bit Operations/Compare To Constant  SystemSampleTime=-1  relop===  const=0  LogicOutDataTypeMode=uint8
  Constant : Constant  OutDataType=fixdt(1, 16)  OutScaling=2^0
  Switch : Switch  Criteria=u2 ~= 0  OutDataType=fixdt(1, 16)  OutScaling=2^0
  PhaseOut : Outport  OutDataType=fixdt(1, 16)  OutScaling=2^0
  wires:
  Constant/1 -> Add/1
  Add/1 -> Switch/1
  Compare To Constant/1 -> Switch/2
  PhaseIn/1 -> Add/2, Switch/3, Compare To Constant/1
  Switch/1 -> PhaseOut/1

== system MyVhclOperator_RTW/MyVhclOperator/Trg: OperState_Driving/OperState_PowerOff/OperState: PowerAcc ==
  note: Operation State:
      | PowerAcc
  GBKind : Inport  OutDataType=fixdt(1, 16)  OutScaling=2^0
  Brake : Constant  Value=0.0  OutDataType=fixdt(1, 16)  OutScaling=2^0
  BrakePark : Constant  Value=1.0  OutDataType=fixdt(1, 16)  OutScaling=2^0
  Bus Creator : BusCreator  Inputs=7
  Bus Creator1 : BusCreator  Inputs=3
  Bus Creator2 : BusCreator  Inputs=3
  Bus Selector : BusSelector  OutputSignals=GearNo,Clutch,SelectorCtrl
  Clutch : Constant  Value=0.0  OutDataType=fixdt(1, 16)  OutScaling=2^0
  GBKind_Manual : simulink/Logic and Bit Operations/Compare To Constant  SystemSampleTime=-1  relop===  const=1  LogicOutDataTypeMode=uint8
  Gas : Constant  Value=0.0  OutDataType=fixdt(1, 16)  OutScaling=2^0
  GearNo : Constant  Value=0  OutDataType=fixdt(1, 16)  OutScaling=2^0
  KeyPos_KeyIn_PowerAcc : Constant  Value=2  OutDataType=fixdt(1, 16)  OutScaling=2^0
  No_Clutch : Constant  Value=0.0  OutDataType=fixdt(1, 16)  OutScaling=2^0
  No_GearNo : Constant  Value=0  OutDataType=fixdt(1, 16)  OutScaling=2^0
  No_SelectorCtrl : Constant  Value=0  OutDataType=fixdt(1, 16)  OutScaling=2^0
  SelectorCtrl_P : Constant  Value=-9  OutDataType=fixdt(1, 16)  OutScaling=2^0
  Switch : Switch  Criteria=u2 ~= 0  OutDataType=fixdt(1, 16)  OutScaling=2^0
  BusOut : Outport  OutDataType=fixdt(1, 16)  OutScaling=2^0
  wires:
  GBKind_Manual/1 -> Switch/2
  GBKind/1 -> GBKind_Manual/1
  Bus Creator2/1 -> Switch/3
  SelectorCtrl_P/1 -> Bus Creator2/3  "SelectorCtrl"
  No_Clutch/1 -> Bus Creator2/2  "Clutch"
  No_GearNo/1 -> Bus Creator2/1  "GearNo"
  No_SelectorCtrl/1 -> Bus Creator1/3  "SelectorCtrl"
  Clutch/1 -> Bus Creator1/2  "Clutch"
  GearNo/1 -> Bus Creator1/1  "GearNo"
  Bus Creator1/1 -> Switch/1
  Switch/1 -> Bus Selector/1
  BrakePark/1 -> Bus Creator/7  "BrakePark"
  Brake/1 -> Bus Creator/6  "Brake"
  Gas/1 -> Bus Creator/5  "Gas"
  KeyPos_KeyIn_PowerAcc/1 -> Bus Creator/4  "Key"
  Bus Selector/3 -> Bus Creator/3  "<SelectorCtrl>"
  Bus Selector/2 -> Bus Creator/2  "<Clutch>"
  Bus Selector/1 -> Bus Creator/1  "<GearNo>"
  Bus Creator/1 -> BusOut/1

== system MyVhclOperator_RTW/MyVhclOperator/Trg: OperState_Driving/OperState_PowerOff/SetOutputAndWait ==
  PhaseIn : Inport  OutDataType=fixdt(1, 16)  OutScaling=2^0
  Add : Sum  OutDataType=fixdt(1, 16)  OutScaling=2^-10
  Compare To Constant : simulink/Logic and Bit Operations/Compare To Constant  SystemSampleTime=-1  relop===  const=0  LogicOutDataTypeMode=uint8
  Constant : Constant  OutDataType=fixdt(1, 16)  OutScaling=2^0
  Switch : Switch  Criteria=u2 ~= 0  OutDataType=fixdt(1, 16)  OutScaling=2^0
  PhaseOut : Outport  OutDataType=fixdt(1, 16)  OutScaling=2^0
  wires:
  Switch/1 -> PhaseOut/1
  PhaseIn/1 -> Compare To Constant/1, Switch/3, Add/2
  Compare To Constant/1 -> Switch/2
  Add/1 -> Switch/1
  Constant/1 -> Add/1

== system MyVhclOperator_RTW/MyVhclOperator/Trg: OperState_Driving/OperState_PowerOn/OperState: Starting ==
  note: Operation State:
      | Starting
  GBKind : Inport  OutDataType=fixdt(1, 16)  OutScaling=2^0
  Brake : Constant  Value=1.0  OutDataType=fixdt(1, 16)  OutScaling=2^0
  BrakePark : Constant  Value=0.0  OutDataType=fixdt(1, 16)  OutScaling=2^0
  Bus Creator : BusCreator  Inputs=7
  Bus Creator1 : BusCreator  Inputs=3
  Bus Creator2 : BusCreator  Inputs=3
  Bus Selector : BusSelector  OutputSignals=GearNo,Clutch,SelectorCtrl
  Clutch : Constant  Value=1.0  OutDataType=fixdt(1, 16)  OutScaling=2^0
  GBKind_Manual : simulink/Logic and Bit Operations/Compare To Constant  SystemSampleTime=-1  relop===  const=1  LogicOutDataTypeMode=uint8
  Gas : Constant  Value=0.0  OutDataType=fixdt(1, 16)  OutScaling=2^0
  GearNo : Constant  Value=0  OutDataType=fixdt(1, 16)  OutScaling=2^0
  KeyPos_KeyIn_Starter : Constant  Value=4  OutDataType=fixdt(1, 16)  OutScaling=2^0
  No_Clutch : Constant  Value=0.0  OutDataType=fixdt(1, 16)  OutScaling=2^0
  No_GearNo : Constant  Value=0  OutDataType=fixdt(1, 16)  OutScaling=2^0
  No_SelectorCtrl : Constant  Value=0  OutDataType=fixdt(1, 16)  OutScaling=2^0
  SelectorCtrl_N : Constant  Value=0  OutDataType=fixdt(1, 16)  OutScaling=2^0
  Switch : Switch  Criteria=u2 ~= 0  OutDataType=fixdt(1, 16)  OutScaling=2^0
  BusOut : Outport  OutDataType=fixdt(1, 16)  OutScaling=2^0
  wires:
  GBKind_Manual/1 -> Switch/2
  GBKind/1 -> GBKind_Manual/1
  Bus Creator2/1 -> Switch/3
  SelectorCtrl_N/1 -> Bus Creator2/3  "SelectorCtrl"
  No_Clutch/1 -> Bus Creator2/2  "Clutch"
  No_GearNo/1 -> Bus Creator2/1  "GearNo"
  No_SelectorCtrl/1 -> Bus Creator1/3  "SelectorCtrl"
  Clutch/1 -> Bus Creator1/2  "Clutch"
  GearNo/1 -> Bus Creator1/1  "GearNo"
  Bus Creator1/1 -> Switch/1
  Switch/1 -> Bus Selector/1
  BrakePark/1 -> Bus Creator/7  "BrakePark"
  Brake/1 -> Bus Creator/6  "Brake"
  Gas/1 -> Bus Creator/5  "Gas"
  KeyPos_KeyIn_Starter/1 -> Bus Creator/4  "Key"
  Bus Selector/3 -> Bus Creator/3  "<SelectorCtrl>"
  Bus Selector/2 -> Bus Creator/2  "<Clutch>"
  Bus Selector/1 -> Bus Creator/1  "<GearNo>"
  Bus Creator/1 -> BusOut/1

== system MyVhclOperator_RTW/MyVhclOperator/Trg: OperState_Driving/OperState_PowerOn/SetOutputAndWait ==
  PhaseIn : Inport  OutDataType=fixdt(1, 16)  OutScaling=2^0
  Add : Sum  OutDataType=fixdt(1, 16)  OutScaling=2^-10
  Compare To Constant : simulink/Logic and Bit Operations/Compare To Constant  SystemSampleTime=-1  relop===  const=0  LogicOutDataTypeMode=uint8
  Constant : Constant  OutDataType=fixdt(1, 16)  OutScaling=2^0
  Switch : Switch  Criteria=u2 ~= 0  OutDataType=fixdt(1, 16)  OutScaling=2^0
  PhaseOut : Outport  OutDataType=fixdt(1, 16)  OutScaling=2^0
  wires:
  Constant/1 -> Add/1
  Add/1 -> Switch/1
  Compare To Constant/1 -> Switch/2
  PhaseIn/1 -> Add/2, Switch/3, Compare To Constant/1
  Switch/1 -> PhaseOut/1

== system MyVhclOperator_RTW/MyVhclOperator/Trg: OperState_PowerOff/OperState_Absent/OperState: PowerOff ==
  note: Operation State:
      | PowerOff
  GBKind : Inport  OutDataType=fixdt(1, 16)  OutScaling=2^0
  Brake : Constant  Value=0.0  OutDataType=fixdt(1, 16)  OutScaling=2^0
  BrakePark : Constant  Value=1.0  OutDataType=fixdt(1, 16)  OutScaling=2^0
  Bus Creator : BusCreator  Inputs=7
  Bus Creator1 : BusCreator  Inputs=3
  Bus Creator2 : BusCreator  Inputs=3
  Bus Selector : BusSelector  OutputSignals=GearNo,Clutch,SelectorCtrl
  Clutch : Constant  Value=0.0  OutDataType=fixdt(1, 16)  OutScaling=2^0
  GBKind_Manual : simulink/Logic and Bit Operations/Compare To Constant  SystemSampleTime=-1  relop===  const=1  LogicOutDataTypeMode=uint8
  Gas : Constant  Value=0.0  OutDataType=fixdt(1, 16)  OutScaling=2^0
  GearNo : Constant  Value=0  OutDataType=fixdt(1, 16)  OutScaling=2^0
  KeyPos_KeyIn_PowerOff : Constant  OutDataType=fixdt(1, 16)  OutScaling=2^0
  No_Clutch : Constant  Value=0.0  OutDataType=fixdt(1, 16)  OutScaling=2^0
  No_GearNo : Constant  Value=0  OutDataType=fixdt(1, 16)  OutScaling=2^0
  No_SelectorCtrl : Constant  Value=0  OutDataType=fixdt(1, 16)  OutScaling=2^0
  SelectorCtrl_P : Constant  Value=-9  OutDataType=fixdt(1, 16)  OutScaling=2^0
  Switch : Switch  Criteria=u2 ~= 0  OutDataType=fixdt(1, 16)  OutScaling=2^0
  BusOut : Outport  OutDataType=fixdt(1, 16)  OutScaling=2^0
  wires:
  GBKind_Manual/1 -> Switch/2
  GBKind/1 -> GBKind_Manual/1
  Bus Creator2/1 -> Switch/3
  SelectorCtrl_P/1 -> Bus Creator2/3  "SelectorCtrl"
  No_Clutch/1 -> Bus Creator2/2  "Clutch"
  No_GearNo/1 -> Bus Creator2/1  "GearNo"
  No_SelectorCtrl/1 -> Bus Creator1/3  "SelectorCtrl"
  Clutch/1 -> Bus Creator1/2  "Clutch"
  GearNo/1 -> Bus Creator1/1  "GearNo"
  Bus Creator1/1 -> Switch/1
  Switch/1 -> Bus Selector/1
  BrakePark/1 -> Bus Creator/7  "BrakePark"
  Brake/1 -> Bus Creator/6  "Brake"
  Gas/1 -> Bus Creator/5  "Gas"
  KeyPos_KeyIn_PowerOff/1 -> Bus Creator/4  "Key"
  Bus Selector/3 -> Bus Creator/3  "<SelectorCtrl>"
  Bus Selector/2 -> Bus Creator/2  "<Clutch>"
  Bus Selector/1 -> Bus Creator/1  "<GearNo>"
  Bus Creator/1 -> BusOut/1

== system MyVhclOperator_RTW/MyVhclOperator/Trg: OperState_PowerOff/OperState_Driving/Drive2Off ==
  note: Drive2Off
  BusIn : Inport  OutDataType=fixdt(1, 16)  OutScaling=2^0
  Active Brake : Subsystem  TreatAsAtomicUnit=on
  Brake to standstill? : Subsystem  TreatAsAtomicUnit=on
  Bus Selector : BusSelector  OutputSignals=Phase
  BusIn_Copy : InportShadow  Port=1  OutDataType=fixdt(1, 16)  OutScaling=2^0
  Key PowerOff : Subsystem  TreatAsAtomicUnit=on
  Merge : Merge  Inputs=5
  Switch Case : SwitchCase  CaseConditions={0,1,2,3,4}  ShowDefaultCase=off
  Wait for PowerOff : Subsystem  TreatAsAtomicUnit=on
  Wait until Standstill : Subsystem  TreatAsAtomicUnit=on
  BusOut : Outport  OutDataType=fixdt(1, 16)  OutScaling=2^0
  wires:
  Bus Selector/1 -> Switch Case/1  "<Phase>"
  Wait for PowerOff/1(BusOut) -> Merge/5
  Key PowerOff/1(BusOut) -> Merge/4
  Wait until Standstill/1(BusOut) -> Merge/3
  Active Brake/1(BusOut) -> Merge/2
  Brake to standstill?/1(BusOut) -> Merge/1
  BusIn_Copy/1 -> Brake to standstill?/1(BusIn), Active Brake/1(BusIn), Wait until Standstill/1(BusIn), Key PowerOff/1(BusIn), Wait for PowerOff/1(BusIn)
  Switch Case/5 -> Wait for PowerOff/Action
  Switch Case/4 -> Key PowerOff/Action
  Switch Case/3 -> Wait until Standstill/Action
  Merge/1 -> BusOut/1
  Switch Case/2 -> Active Brake/Action
  Switch Case/1 -> Brake to standstill?/Action
  BusIn/1 -> Bus Selector/1

== system MyVhclOperator_RTW/MyVhclOperator/Trg: OperState_PowerOff/OperState_PowerAccessory/OperState: PowerOn ==
  note: Operation State:
      | PowerOn
  GBKind : Inport  OutDataType=fixdt(1, 16)  OutScaling=2^0
  Brake : Constant  Value=0.0  OutDataType=fixdt(1, 16)  OutScaling=2^0
  BrakePark : Constant  Value=1.0  OutDataType=fixdt(1, 16)  OutScaling=2^0
  Bus Creator : BusCreator  Inputs=7
  Bus Creator1 : BusCreator  Inputs=3
  Bus Creator2 : BusCreator  Inputs=3
  Bus Selector : BusSelector  OutputSignals=GearNo,Clutch,SelectorCtrl
  Clutch : Constant  Value=0.0  OutDataType=fixdt(1, 16)  OutScaling=2^0
  GBKind_Manual : simulink/Logic and Bit Operations/Compare To Constant  SystemSampleTime=-1  relop===  const=1  LogicOutDataTypeMode=uint8
  Gas : Constant  Value=0.0  OutDataType=fixdt(1, 16)  OutScaling=2^0
  GearNo : Constant  Value=0  OutDataType=fixdt(1, 16)  OutScaling=2^0
  KeyPos_KeyIn_PowerOn : Constant  Value=3  OutDataType=fixdt(1, 16)  OutScaling=2^0
  No_Clutch : Constant  Value=0.0  OutDataType=fixdt(1, 16)  OutScaling=2^0
  No_GearNo : Constant  Value=0  OutDataType=fixdt(1, 16)  OutScaling=2^0
  No_SelectorCtrl : Constant  Value=0  OutDataType=fixdt(1, 16)  OutScaling=2^0
  SelectorCtrl_P : Constant  Value=-9  OutDataType=fixdt(1, 16)  OutScaling=2^0
  Switch : Switch  Criteria=u2 ~= 0  OutDataType=fixdt(1, 16)  OutScaling=2^0
  BusOut : Outport  OutDataType=fixdt(1, 16)  OutScaling=2^0
  wires:
  Bus Creator/1 -> BusOut/1
  Bus Selector/1 -> Bus Creator/1  "<GearNo>"
  Bus Selector/2 -> Bus Creator/2  "<Clutch>"
  Bus Selector/3 -> Bus Creator/3  "<SelectorCtrl>"
  KeyPos_KeyIn_PowerOn/1 -> Bus Creator/4  "Key"
  Gas/1 -> Bus Creator/5  "Gas"
  Brake/1 -> Bus Creator/6  "Brake"
  BrakePark/1 -> Bus Creator/7  "BrakePark"
  Switch/1 -> Bus Selector/1
  Bus Creator1/1 -> Switch/1
  GearNo/1 -> Bus Creator1/1  "GearNo"
  Clutch/1 -> Bus Creator1/2  "Clutch"
  No_SelectorCtrl/1 -> Bus Creator1/3  "SelectorCtrl"
  No_GearNo/1 -> Bus Creator2/1  "GearNo"
  No_Clutch/1 -> Bus Creator2/2  "Clutch"
  SelectorCtrl_P/1 -> Bus Creator2/3  "SelectorCtrl"
  Bus Creator2/1 -> Switch/3
  GBKind/1 -> GBKind_Manual/1
  GBKind_Manual/1 -> Switch/2

== system MyVhclOperator_RTW/MyVhclOperator/Trg: OperState_PowerOff/OperState_PowerAccessory/SetOutputAndWait ==
  PhaseIn : Inport  OutDataType=fixdt(1, 16)  OutScaling=2^0
  Add : Sum  OutDataType=fixdt(1, 16)  OutScaling=2^-10
  Compare To Constant : simulink/Logic and Bit Operations/Compare To Constant  SystemSampleTime=-1  relop===  const=0  LogicOutDataTypeMode=uint8
  Constant : Constant  OutDataType=fixdt(1, 16)  OutScaling=2^0
  Switch : Switch  Criteria=u2 ~= 0  OutDataType=fixdt(1, 16)  OutScaling=2^0
  PhaseOut : Outport  OutDataType=fixdt(1, 16)  OutScaling=2^0
  wires:
  Switch/1 -> PhaseOut/1
  PhaseIn/1 -> Compare To Constant/1, Switch/3, Add/2
  Compare To Constant/1 -> Switch/2
  Add/1 -> Switch/1
  Constant/1 -> Add/1

== system MyVhclOperator_RTW/MyVhclOperator/Trg: OperState_PowerOff/OperState_PowerOff/OperState: PowerOff ==
  note: Operation State:
      | PowerOff
  GBKind : Inport  OutDataType=fixdt(1, 16)  OutScaling=2^0
  Brake : Constant  Value=0.0  OutDataType=fixdt(1, 16)  OutScaling=2^0
  BrakePark : Constant  Value=1.0  OutDataType=fixdt(1, 16)  OutScaling=2^0
  Bus Creator : BusCreator  Inputs=7
  Bus Creator1 : BusCreator  Inputs=3
  Bus Creator2 : BusCreator  Inputs=3
  Bus Selector : BusSelector  OutputSignals=GearNo,Clutch,SelectorCtrl
  Clutch : Constant  Value=0.0  OutDataType=fixdt(1, 16)  OutScaling=2^0
  GBKind_Manual : simulink/Logic and Bit Operations/Compare To Constant  SystemSampleTime=-1  relop===  const=1  LogicOutDataTypeMode=uint8
  Gas : Constant  Value=0.0  OutDataType=fixdt(1, 16)  OutScaling=2^0
  GearNo : Constant  Value=0  OutDataType=fixdt(1, 16)  OutScaling=2^0
  KeyPos_KeyIn_PowerOff : Constant  OutDataType=fixdt(1, 16)  OutScaling=2^0
  No_Clutch : Constant  Value=0.0  OutDataType=fixdt(1, 16)  OutScaling=2^0
  No_GearNo : Constant  Value=0  OutDataType=fixdt(1, 16)  OutScaling=2^0
  No_SelectorCtrl : Constant  Value=0  OutDataType=fixdt(1, 16)  OutScaling=2^0
  SelectorCtrl_P : Constant  Value=-9  OutDataType=fixdt(1, 16)  OutScaling=2^0
  Switch : Switch  Criteria=u2 ~= 0  OutDataType=fixdt(1, 16)  OutScaling=2^0
  BusOut : Outport  OutDataType=fixdt(1, 16)  OutScaling=2^0
  wires:
  GBKind_Manual/1 -> Switch/2
  GBKind/1 -> GBKind_Manual/1
  Bus Creator2/1 -> Switch/3
  SelectorCtrl_P/1 -> Bus Creator2/3  "SelectorCtrl"
  No_Clutch/1 -> Bus Creator2/2  "Clutch"
  No_GearNo/1 -> Bus Creator2/1  "GearNo"
  No_SelectorCtrl/1 -> Bus Creator1/3  "SelectorCtrl"
  Clutch/1 -> Bus Creator1/2  "Clutch"
  GearNo/1 -> Bus Creator1/1  "GearNo"
  Bus Creator1/1 -> Switch/1
  Switch/1 -> Bus Selector/1
  BrakePark/1 -> Bus Creator/7  "BrakePark"
  Brake/1 -> Bus Creator/6  "Brake"
  Gas/1 -> Bus Creator/5  "Gas"
  KeyPos_KeyIn_PowerOff/1 -> Bus Creator/4  "Key"
  Bus Selector/3 -> Bus Creator/3  "<SelectorCtrl>"
  Bus Selector/2 -> Bus Creator/2  "<Clutch>"
  Bus Selector/1 -> Bus Creator/1  "<GearNo>"
  Bus Creator/1 -> BusOut/1

== system MyVhclOperator_RTW/MyVhclOperator/Trg: OperState_PowerOff/OperState_PowerOn/OperState: PowerOff ==
  note: Operation State:
      | PowerOff
  GBKind : Inport  OutDataType=fixdt(1, 16)  OutScaling=2^0
  Brake : Constant  Value=0.0  OutDataType=fixdt(1, 16)  OutScaling=2^0
  BrakePark : Constant  Value=1.0  OutDataType=fixdt(1, 16)  OutScaling=2^0
  Bus Creator : BusCreator  Inputs=7
  Bus Creator1 : BusCreator  Inputs=3
  Bus Creator2 : BusCreator  Inputs=3
  Bus Selector : BusSelector  OutputSignals=GearNo,Clutch,SelectorCtrl
  Clutch : Constant  Value=0.0  OutDataType=fixdt(1, 16)  OutScaling=2^0
  GBKind_Manual : simulink/Logic and Bit Operations/Compare To Constant  SystemSampleTime=-1  relop===  const=1  LogicOutDataTypeMode=uint8
  Gas : Constant  Value=0.0  OutDataType=fixdt(1, 16)  OutScaling=2^0
  GearNo : Constant  Value=0  OutDataType=fixdt(1, 16)  OutScaling=2^0
  KeyPos_KeyIn_PowerOff : Constant  OutDataType=fixdt(1, 16)  OutScaling=2^0
  No_Clutch : Constant  Value=0.0  OutDataType=fixdt(1, 16)  OutScaling=2^0
  No_GearNo : Constant  Value=0  OutDataType=fixdt(1, 16)  OutScaling=2^0
  No_SelectorCtrl : Constant  Value=0  OutDataType=fixdt(1, 16)  OutScaling=2^0
  SelectorCtrl_P : Constant  Value=-9  OutDataType=fixdt(1, 16)  OutScaling=2^0
  Switch : Switch  Criteria=u2 ~= 0  OutDataType=fixdt(1, 16)  OutScaling=2^0
  BusOut : Outport  OutDataType=fixdt(1, 16)  OutScaling=2^0
  wires:
  Bus Creator/1 -> BusOut/1
  Bus Selector/1 -> Bus Creator/1  "<GearNo>"
  Bus Selector/2 -> Bus Creator/2  "<Clutch>"
  Bus Selector/3 -> Bus Creator/3  "<SelectorCtrl>"
  KeyPos_KeyIn_PowerOff/1 -> Bus Creator/4  "Key"
  Gas/1 -> Bus Creator/5  "Gas"
  Brake/1 -> Bus Creator/6  "Brake"
  BrakePark/1 -> Bus Creator/7  "BrakePark"
  Switch/1 -> Bus Selector/1
  Bus Creator1/1 -> Switch/1
  GearNo/1 -> Bus Creator1/1  "GearNo"
  Clutch/1 -> Bus Creator1/2  "Clutch"
  No_SelectorCtrl/1 -> Bus Creator1/3  "SelectorCtrl"
  No_GearNo/1 -> Bus Creator2/1  "GearNo"
  No_Clutch/1 -> Bus Creator2/2  "Clutch"
  SelectorCtrl_P/1 -> Bus Creator2/3  "SelectorCtrl"
  Bus Creator2/1 -> Switch/3
  GBKind/1 -> GBKind_Manual/1
  GBKind_Manual/1 -> Switch/2

== system MyVhclOperator_RTW/MyVhclOperator/Trg: OperState_PowerOff/OperState_PowerOn/SetOutputAndWait ==
  PhaseIn : Inport  OutDataType=fixdt(1, 16)  OutScaling=2^0
  Add : Sum  OutDataType=fixdt(1, 16)  OutScaling=2^-10
  Compare To Constant : simulink/Logic and Bit Operations/Compare To Constant  SystemSampleTime=-1  relop===  const=0  LogicOutDataTypeMode=uint8
  Constant : Constant  OutDataType=fixdt(1, 16)  OutScaling=2^0
  Switch : Switch  Criteria=u2 ~= 0  OutDataType=fixdt(1, 16)  OutScaling=2^0
  PhaseOut : Outport  OutDataType=fixdt(1, 16)  OutScaling=2^0
  wires:
  Constant/1 -> Add/1
  Add/1 -> Switch/1
  Compare To Constant/1 -> Switch/2
  PhaseIn/1 -> Add/2, Switch/3, Compare To Constant/1
  Switch/1 -> PhaseOut/1
